simulink model "TempCtrlClosedLoop_SIL"  (R2026a)
settings: Solver=ode3  StopTime=inf  FixedStep=0.005
InitFcn:
  | % Interface bus objects of temp controller FMU (TcIn/TcOut); fixed names so the model is self-contained
  | e=Simulink.BusElement; e.Name='Temp'; e.DataType='int16'; b=Simulink.Bus; b.Elements=e; TcIn_TempCtrlSysPT2=b;
  | e=Simulink.BusElement; e.Name='setpoint'; e.DataType='double'; b=Simulink.Bus; b.Elements=e; e=Simulink.BusElement; e.Name='actual'; e.DataType='double'; b.Elements(2)=e; MonitoringSignalsType=b;
  | e=Simulink.BusElement; e.Name='Heat_On'; e.DataType='boolean'; b=Simulink.Bus; b.Elements=e; e=Simulink.BusElement; e.Name='MonitoringSignals'; e.DataType='Bus: MonitoringSignalsType'; b.Elements(2)=e; TcOut_TempCtrlSysPT2=b;
  | e=Simulink.BusElement; e.Name='TempCtrlSysPT2'; e.DataType='Bus: TcIn_TempCtrlSysPT2'; b=Simulink.Bus; b.Elements=e; TcIn=b;
  | e=Simulink.BusElement; e.Name='TempCtrlSysPT2'; e.DataType='Bus: TcOut_TempCtrlSysPT2'; b=Simulink.Bus; b.Elements=e; TcOut=b;
  | clear e b
settings Model: Creator=MatthiasJ  LastModifiedBy=Admin
settings DataIOCC: SignalLoggingSaveFormat=ModelDataLogs
settings OptimizationCC: LocalBlockOutputs=off
settings DebuggingCC: UnderspecifiedInitializationDetection=Classic
settings HardwareCC: ProdHWDeviceType=32-bit Generic
settings SFSimCC: SimTargetLang=C++
settings RTWCC: GenCodeOnly=on  GenerateReport=on  RTWVerbose=off  RetainRTWFile=on  TargetLang=C++
settings CodeAppCC: MaxIdLength=50.0
settings GRTTargetCC: CodeInterfacePackaging=C++ class  SubcomponentCodeInterfacePackaging=C++ class

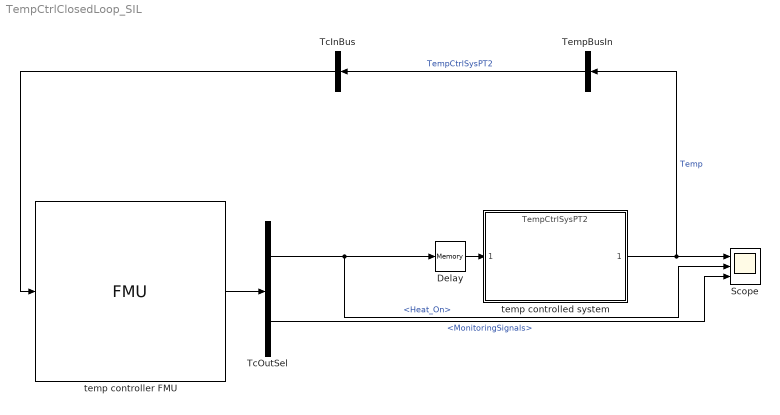
== system TempCtrlClosedLoop_SIL ==
  Delay : Memory
  Scope : Scope  NumInputPorts=3
      settings: TimeSpan=10  ActiveDisplayYMinimum=168.75  ActiveDisplayYMaximum=481.25
  TcInBus : BusCreator  Inputs=1  OutDataTypeStr=Bus: TcIn  NonVirtualBus=on
  TcOutSel : BusSelector  OutputSignals=TempCtrlSysPT2.Heat_On,TempCtrlSysPT2.MonitoringSignals
  TempBusIn : BusCreator  Inputs=1  OutDataTypeStr=Bus: TcIn_TempCtrlSysPT2
  temp controlled system : ModelReference  ModelNameDialog=TempCtrlSysPT2  ModelReferenceVersion=17.7
  temp controller FMU : FMU  FMUName=TcSimRuntimeTempCtrl.fmu  FMUMode=CoSimulation  FMUInitializeEnumObject=off
      mask Type: TcSimRuntimeFmi [Co-Simulation, v3.0]
      mask Display:
      | if (exist([Simulink.fileGenControl('get','CacheFolder') '\slprj\_fmu\aa7c3491d863e6540a18b5d4246446ba\TcSimRuntimeTempCtrl\terminalsAndIcons\icon.svg'],'file'))
      |     image([Simulink.fileGenControl('get','CacheFolder') '\slprj\_fmu\aa7c3491d863e6540a18b5d4246446ba\TcSimRuntimeTempCtrl\terminalsAndIcons\icon.svg']);
      | else
      |     disp('TcSimRuntimeFmi [Co-Simulation, v3.0]');
      | end
      | port_label('output',1,'TcOut');
      | port_label('input',1,'TcIn');
  wires:
  Delay/1 -> temp controlled system/1
  temp controller FMU/1 -> TcOutSel/1
  TcOutSel/1 -> Scope/2, Delay/1  "<Heat_On>"
  TcInBus/1 -> temp controller FMU/1
  TempBusIn/1 -> TcInBus/1  "TempCtrlSysPT2"
  temp controlled system/1 -> TempBusIn/1, Scope/1  "Temp"
  TcOutSel/2 -> Scope/3  "<MonitoringSignals>"
